simulink model "model1"  (R2025a)
settings: Solver=FixedStepAuto  StartTime=0.0  StopTime=3600  FixedStep=1  RelTol=1e-3
libraries: fuzblock x3
settings Model: Creator=boris  LastModifiedBy=Matija Leković

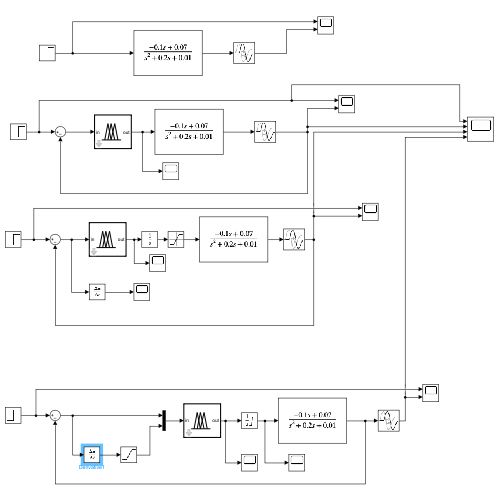
[thumbnail: Simulink's stored preview of the top-level diagram]
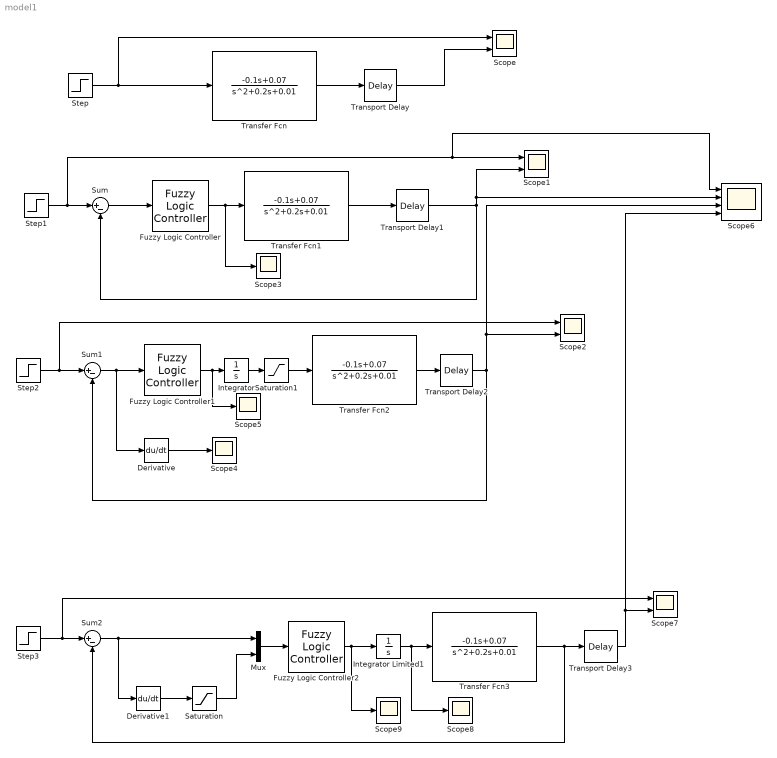
== system model1 ==
  Derivative : Derivative
  Derivative1 : Derivative
  Fuzzy Logic Controller : fuzblock/Fuzzy Logic  Controller  FIS='prviprvasema.fis'  OutputSampleNumber=101  DataType=double  UseLookupTable=off  NumBreakpoints=10  FuzzifiedInputs=off  RuleFiringStrengths=off  RuleOutputs=off  AggregatedOutputs=off  SimulateUsing=Interpreted execution  OutOfRangeInputValueMessage=warning  NoRuleFiredMessage=warning  EmptyOutputFuzzySetMessage=warning
  Fuzzy Logic Controller1 : fuzblock/Fuzzy Logic  Controller  FIS='prviprvasema.fis'  OutputSampleNumber=101  DataType=double  UseLookupTable=off  NumBreakpoints=10  FuzzifiedInputs=off  RuleFiringStrengths=off  RuleOutputs=off  AggregatedOutputs=off  SimulateUsing=Interpreted execution  OutOfRangeInputValueMessage=warning  NoRuleFiredMessage=warning  EmptyOutputFuzzySetMessage=warning
  Fuzzy Logic Controller2 : fuzblock/Fuzzy Logic  Controller  FIS='prvidrugasema.fis'  OutputSampleNumber=101  DataType=double  UseLookupTable=off  NumBreakpoints=10  FuzzifiedInputs=off  RuleFiringStrengths=off  RuleOutputs=off  AggregatedOutputs=off  SimulateUsing=Interpreted execution  OutOfRangeInputValueMessage=warning  NoRuleFiredMessage=warning  EmptyOutputFuzzySetMessage=warning
  Integrator : Integrator
  Integrator Limited1 : Integrator  LimitOutput=on  UpperSaturationLimit=1  LowerSaturationLimit=-1
  Mux : Mux  Inputs=2
  Saturation : Saturate
  Saturation1 : Saturate  UpperLimit=1  LowerLimit=-1
  Scope{,1..2,7} (4 alike) : Scope  NumInputPorts=2
      Scope settings: ActiveDisplayYMinimum=-12.396957084882809  ActiveDisplayYMaximum=10.479794503636402
      Scope1 settings: ActiveDisplayYMinimum=-2.5  ActiveDisplayYMaximum=2.5
      Scope2 settings: ActiveDisplayYMinimum=-10.086533195257967  ActiveDisplayYMaximum=11.700849269998422  DataLoggingVariableName=ScopeData2
      Scope7 settings: ActiveDisplayYMinimum=-3.8971576169763207  ActiveDisplayYMaximum=4.9492969260875377  DataLoggingVariableName=ScopeData7
  Scope{3..5,8..9} (5 alike) : Scope
      Scope3 settings: ActiveDisplayYMinimum=-1  ActiveDisplayYMaximum=1  DataLoggingVariableName=ScopeData3
      Scope4 settings: ActiveDisplayYMinimum=-1.0074504598282843  ActiveDisplayYMaximum=4.0466985831125815  DataLoggingVariableName=ScopeData4
      Scope5 settings: ActiveDisplayYMinimum=-2.0101596281485179  ActiveDisplayYMaximum=1.3731398755799131  DataLoggingVariableName=ScopeData5
      Scope8 settings: ActiveDisplayYMinimum=-1.5490967363861226  ActiveDisplayYMaximum=2.4337970069535433  DataLoggingVariableName=ScopeData8
      Scope9 settings: ActiveDisplayYMinimum=-0.0808683820870154  ActiveDisplayYMaximum=0.0799296911830963  DataLoggingVariableName=ScopeData9
  Scope6 : Scope  NumInputPorts=4
      settings: ActiveDisplayYMinimum=-7.7729712840065019  ActiveDisplayYMaximum=7.8358989546148381  DataLoggingVariableName=ScopeData6
  Step : Step  Time=15*60  Before=-1  SampleTime=0
  Step1 : Step  Time=15*60  Before=-2  After=2  SampleTime=0
  Step2 : Step  Time=15*60  Before=-2  After=2  SampleTime=0
  Step3 : Step  Time=500  Before=-2  After=2  SampleTime=0
  Sum : Sum  Inputs=|+-
  Sum1 : Sum  Inputs=|+-
  Sum2 : Sum  Inputs=|+-
  Transfer Fcn{,1..3} (4 alike) : TransferFcn  Numerator=[-0.1 0.07]  Denominator=[1 0.2 0.01]
  Transport Delay{,1..3} (4 alike) : TransportDelay  DelayTime=3
  wires:
  Step/1 -> Scope/1, Transfer Fcn/1
  Transfer Fcn/1 -> Transport Delay/1
  Transport Delay/1 -> Scope/2
  Transfer Fcn1/1 -> Transport Delay1/1
  Step1/1 -> Sum/1, Scope6/1, Scope1/1
  Sum/1 -> Fuzzy Logic Controller/1
  Fuzzy Logic Controller/1 -> Scope3/1, Transfer Fcn1/1
  Transport Delay1/1 -> Scope1/2, Scope6/2, Sum/2
  Sum1/1 -> Derivative/1, Fuzzy Logic Controller1/1
  Transfer Fcn2/1 -> Transport Delay2/1
  Step2/1 -> Sum1/1, Scope2/1
  Saturation1/1 -> Transfer Fcn2/1
  Fuzzy Logic Controller1/1 -> Scope5/1, Integrator/1
  Derivative/1 -> Scope4/1
  Transport Delay2/1 -> Scope6/3, Scope2/2, Sum1/2
  Fuzzy Logic Controller2/1 -> Scope9/1, Integrator Limited1/1
  Step3/1 -> Sum2/1, Scope7/1
  Transport Delay3/1 -> Scope6/4, Scope7/2
  Transfer Fcn3/1 -> Sum2/2, Transport Delay3/1
  Integrator Limited1/1 -> Scope8/1, Transfer Fcn3/1
  Mux/1 -> Fuzzy Logic Controller2/1
  Derivative1/1 -> Saturation/1
  Sum2/1 -> Mux/1, Derivative1/1
  Saturation/1 -> Mux/2
  Integrator/1 -> Saturation1/1
